simulink model "trajectory_planner"  (R2023a)
settings: Solver=VariableStepAuto  StartTime=0.0  StopTime=60.0  RelTol=1e-3
libraries: shareduavrstlib x1, simulink x1
settings Model: Creator=zhiyu  LastModifiedBy=User

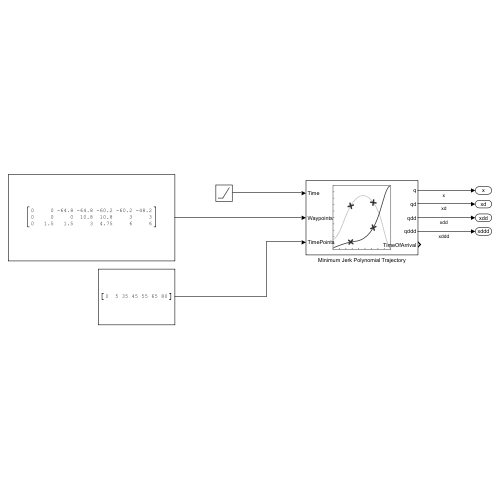
[thumbnail: Simulink's stored preview of the top-level diagram]
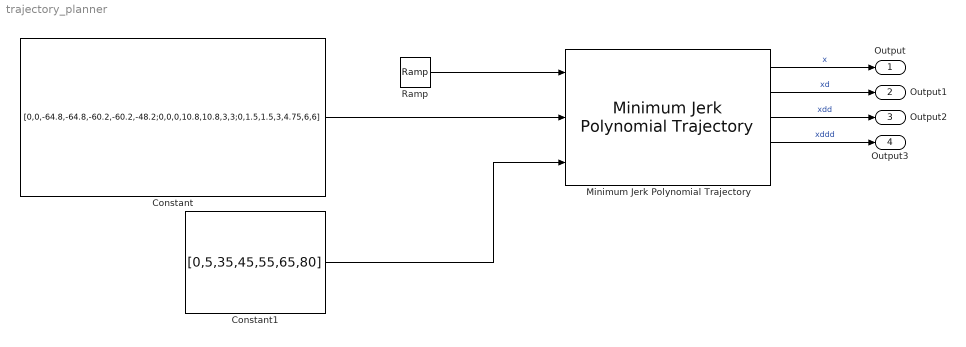
== system trajectory_planner ==
  Constant : Constant  Value=[0,0,-64.8,-64.8,-60.2,-60.2,-48.2;0,0,0,10.8,10.8,3,3;0,1.5,1.5,3,4.75,6,6]  VectorParams1D=off
  Constant1 : Constant  Value=[0,5,35,45,55,65,80]  VectorParams1D=off
  Minimum Jerk Polynomial Trajectory : shareduavrstlib/Minimum Jerk Polynomial Trajectory  ShowBCInputPort=off  ShowPolynomialCoefs=off  ShowStatusOutputPort=off  TimeAllocation=off  TimeWeight=100  MinSegmentTime=0.1  MaxSegmentTime=1  MaxIteration=1500  MaxTime=10  SimulateUsing=Interpreted execution
      settings: LibrarySourceBlock=uavalgslib/Minimum Jerk Polynomial Trajectory
  Ramp : simulink/Sources/Ramp  slope=1  start=0  InitialOutput=0
  Output : Outport
  Output1 : Outport  Port=2
  Output2 : Outport  Port=3
  Output3 : Outport  Port=4
  wires:
  Ramp/1 -> Minimum Jerk Polynomial Trajectory/1
  Constant/1 -> Minimum Jerk Polynomial Trajectory/2
  Constant1/1 -> Minimum Jerk Polynomial Trajectory/3
  Minimum Jerk Polynomial Trajectory/1 -> Output/1  "x"
  Minimum Jerk Polynomial Trajectory/2 -> Output1/1  "xd"
  Minimum Jerk Polynomial Trajectory/3 -> Output2/1  "xdd"
  Minimum Jerk Polynomial Trajectory/4 -> Output3/1  "xddd"
